simulink model "fourmasses_cvxgen"  (Simulink 7.9)
settings: Solver=ode45  StartTime=0.0  StopTime=60  RelTol=1e-3
values from neighbouring files (symbols this model uses):
  A = params.A    [cvxsolve.m]
  B = params.B    [cvxsolve.m]
  dt = 0.5    [prepFourMasses.m]    (also in prepSixMasses.m; prepSoftKS.m)
  Ed_block = Ef_block    [prepFourMasses.m]    (also in prepSixMasses.m; prepSoftKS.m)
  Ef_block = zeros(2*n,1)    [prepFourMasses.m]    (also in prepSixMasses.m; prepSoftKS.m)
  ef_block = Ef_block    [prepFourMasses.m]    (also in prepSixMasses.m; prepSoftKS.m)
  f = params.f    [cvxsolve.m]    (also in prepFourMasses.m = [0.5*ones(4,1)]; prepSixMasses.m = [.5*ones(6,1)]; prepSoftKS.m = [0.5*ones(6,1)])
  Ff = params.Ff    [cvxsolve.m]    (also in prepFourMasses.m = [[1] zeros(1,7)]; prepSixMasses.m = [[1;1] zeros(2,11)]; prepSoftKS.m = [[1;1] zeros(2,11)])
  ff = params.ff    [cvxsolve.m]    (also in prepFourMasses.m = [xmax]; prepSixMasses.m = [.3; .3]; prepSoftKS.m = [.3; .3])
  fs = params.fs    [cvxsolve.m]    (also in prepFourMasses.m = [xmax*ones(4,1) ]*100; prepSixMasses.m = [1*ones(12,1) ]*100; prepSoftKS.m = [0.3*ones(12,1) ]*100)
  Fu = params.Fu    [cvxsolve.m]    (also in prepFourMasses.m = [eye(2); -eye(2) ]; prepSixMasses.m = [eye(3); -eye(3) ]; prepSoftKS.m = [eye(3); -eye(3) ])
  Fus = [zeros(4,2)]    [prepFourMasses.m]    (also in prepSixMasses.m = [zeros(12,3)]; prepSoftKS.m = [zeros(12,3)])
  Fx = [zeros(4,8)]    [prepFourMasses.m]    (also in prepSixMasses.m = [zeros(6,12)]; prepSoftKS.m = [zeros(6,12)])
  Fxs = params.Fxs    [cvxsolve.m]    (also in prepFourMasses.m = [eye(4) zeros(4)]*100; prepSixMasses.m = [eye(6) zeros(6); prepSoftKS.m = [eye(6) zeros(6))
  m = size(B,2)    [prepFourMasses.m]    (also in prepSixMasses.m; prepSoftKS.m)
  n = size(A,1)    [prepFourMasses.m]    (also in prepSixMasses.m; prepSoftKS.m)
  Q = params.Q    [cvxsolve.m]    (also in prepFourMasses.m = eye(8); prepSixMasses.m = eye(12); prepSoftKS.m = eye(12))
  R = params.R    [cvxsolve.m]    (also in prepFourMasses.m = eye(2); prepSixMasses.m = eye(3); prepSoftKS.m = eye(3))
  T = 11    [prepFourMasses.m]    (also in prepSixMasses.m = 31; prepSoftKS.m = 10)
undefined symbols (not defined in the file or in its folder): Qf
settings Model: Creator=aeagr  LastModifiedBy=aeagr

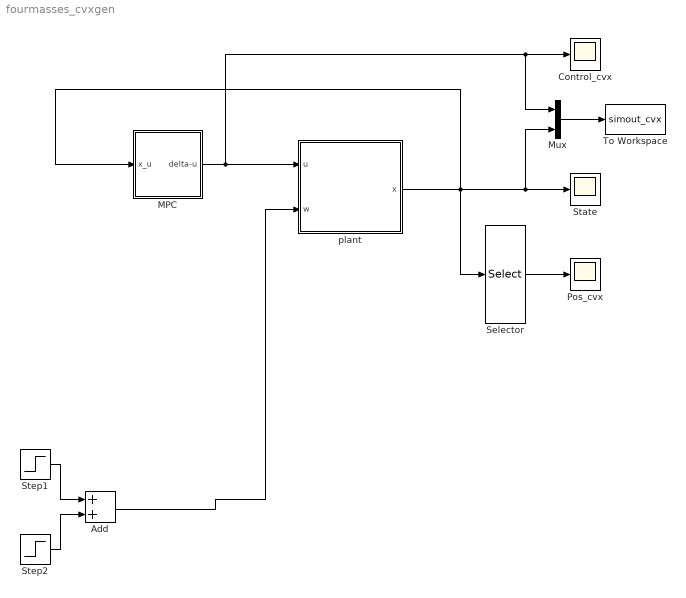
== system fourmasses_cvxgen ==
  Add : Sum
  Control_cvx : Scope
      settings: TimeRange=60  YMin=-0.5  YMax=0.45
  MPC : Subsystem  RequirementInfo={} %GIDa_b6831cb4_84cf_47ee_903b_b1a4a29acb60  TreatAsAtomicUnit=on  SystemSampleTime=dt
      settings: RTWSystemCode=Function  RTWFcnNameOpts=Use subsystem name  RTWFileNameOpts=Use subsystem name
  Mux : Mux  Inputs=2
  Pos_cvx : Scope
      settings: YMin=-0.7  YMax=0.8  SaveName=ScopeData2
  Selector : Selector  InputPortWidth=8  IndexOptions=Index vector (dialog)  Indices=[1:4]  OutputSizes=1
  State : Scope
      settings: YMin=-0.7  YMax=0.8
  Step1 : Step  Time=10  Before=zeros(4,1)  After=[0.5;0;0;0]  SampleTime=0
  Step2 : Step  Time=30  Before=zeros(4,1)  After=-[0.5;0;0;0]  SampleTime=0
  To Workspace : ToWorkspace  VariableName=simout_cvx  SampleTime=-1
  plant : Subsystem
  wires:
  MPC/1(delta-u) -> plant/1(u), Control_cvx/1, Mux/1
  plant/1(x) -> Selector/1, MPC/1(x_u), State/1, Mux/2
  Selector/1 -> Pos_cvx/1
  Add/1 -> plant/2(w)
  Step1/1 -> Add/1
  Step2/1 -> Add/2
  Mux/1 -> To Workspace/1

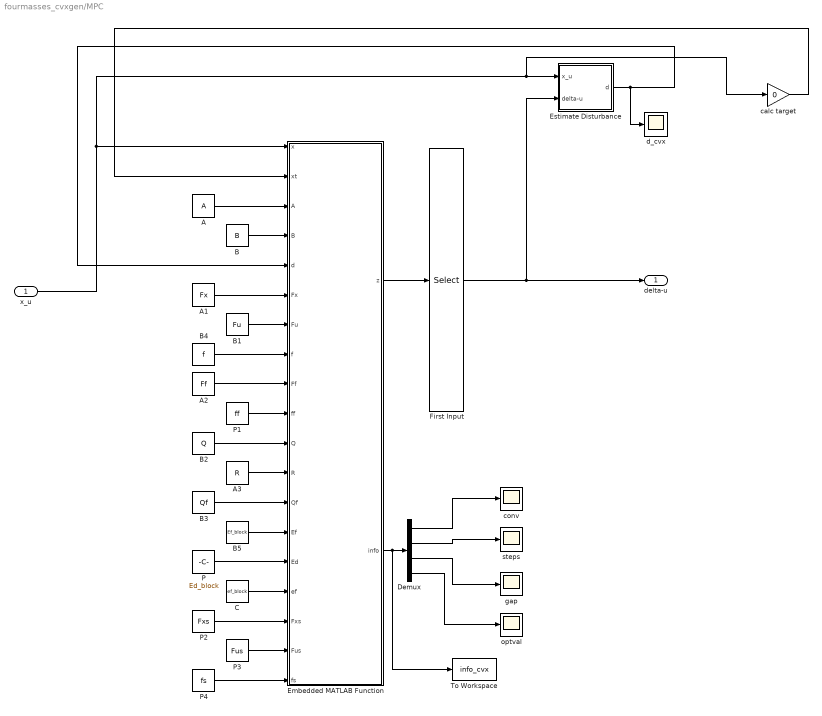
== system fourmasses_cvxgen/MPC ==
  x_u : Inport
  A : Constant  Value=A
  A1 : Constant  Value=Fx
  A2 : Constant  Value=Ff  VectorParams1D=off
  A3 : Constant  Value=R
  B : Constant  Value=B
  B1 : Constant  Value=Fu
  B2 : Constant  Value=Q
  B3 : Constant  Value=Qf
  B4 : Constant  Value=f
  B5 : Constant  Value=Ef_block
  C : Constant  Value=ef_block
  Demux : Demux
  Embedded MATLAB Function : MATLAB Function  TreatAsAtomicUnit=on
      settings: RTWFileNameOpts=Use subsystem name
  Estimate Disturbance : Subsystem
  First Input : Selector  InputPortWidth=T*(n+m)  IndexOptions=Index vector (dialog)  Indices=1:2  OutputSizes=1
  P : Constant  Value=Ed_block
  P1 : Constant  Value=ff
  P2 : Constant  Value=Fxs
  P3 : Constant  Value=Fus
  P4 : Constant  Value=fs
  To Workspace : ToWorkspace  VariableName=info_cvx  SampleTime=-1
  calc target : Gain  Gain=0
  conv : Scope
      settings: YMin=1.65436e-24  YMax=2.75e-08  SaveName=ScopeData3
  d_cvx : Scope
      settings: YMin=-0.00025  YMax=0.002  SaveName=ScopeData6
  gap : Scope
      settings: YMin=1.65436e-24  YMax=2.75e-08  SaveName=ScopeData5
  optval : Scope
      settings: YMin=1.65436e-24  YMax=2.75e-08  SaveName=ScopeData9
  steps : Scope
      settings: YMin=1.65436e-24  YMax=2.75e-08  SaveName=ScopeData4
  delta-u : Outport
  wires:
  First Input/1 -> delta-u/1, Estimate Disturbance/2(delta-u)
  Embedded MATLAB Function/1(z) -> First Input/1
  x_u/1 -> Embedded MATLAB Function/1(x), Estimate Disturbance/1(x_u), calc target/1
  B/1 -> Embedded MATLAB Function/4(B)
  A/1 -> Embedded MATLAB Function/3(A)
  B3/1 -> Embedded MATLAB Function/13(Qf)
  A3/1 -> Embedded MATLAB Function/12(R)
  B2/1 -> Embedded MATLAB Function/11(Q)
  A2/1 -> Embedded MATLAB Function/9(Ff)
  B1/1 -> Embedded MATLAB Function/7(Fu)
  A1/1 -> Embedded MATLAB Function/6(Fx)
  B4/1 -> Embedded MATLAB Function/8(f)
  P1/1 -> Embedded MATLAB Function/10(ff)
  Estimate Disturbance/1(d) -> d_cvx/1, Embedded MATLAB Function/5(d)
  calc target/1 -> Embedded MATLAB Function/2(xt)
  B5/1 -> Embedded MATLAB Function/14(Ef)
  P2/1 -> Embedded MATLAB Function/17(Fxs)
  P3/1 -> Embedded MATLAB Function/18(Fus)
  P/1 -> Embedded MATLAB Function/15(Ed)
  C/1 -> Embedded MATLAB Function/16(ef)
  P4/1 -> Embedded MATLAB Function/19(fs)
  Embedded MATLAB Function/2(info) -> Demux/1, To Workspace/1
  Demux/1 -> conv/1
  Demux/2 -> steps/1
  Demux/3 -> gap/1
  Demux/4 -> optval/1

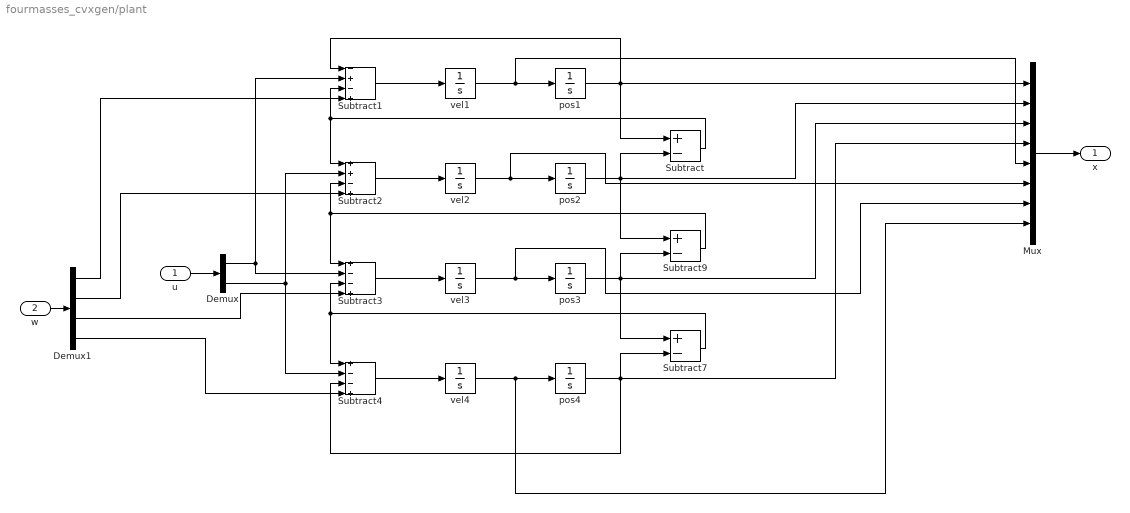
== system fourmasses_cvxgen/plant ==
  u : Inport
  w : Inport  Port=2
  Demux : Demux  Outputs=2
  Demux1 : Demux
  Mux : Mux  Inputs=8
  Subtract : Sum  Inputs=+-
  Subtract1 : Sum  Inputs=-+-+
  Subtract2 : Sum  Inputs=++-+
  Subtract3 : Sum  Inputs=+--+
  Subtract4 : Sum  Inputs=+--+
  Subtract7 : Sum  Inputs=+-
  Subtract9 : Sum  Inputs=+-
  pos{1..4} (4 alike) : Integrator
  vel{1..4} (4 alike) : Integrator
  x : Outport
  wires:
  vel1/1 -> pos1/1, Mux/5
  vel2/1 -> pos2/1, Mux/6
  vel3/1 -> pos3/1, Mux/7
  vel4/1 -> pos4/1, Mux/8
  pos1/1 -> Subtract/1, Subtract1/1, Mux/1
  pos2/1 -> Subtract/2, Subtract9/1, Mux/2
  pos3/1 -> Subtract7/1, Subtract9/2, Mux/3
  pos4/1 -> Subtract7/2, Mux/4, Subtract4/3
  Subtract/1 -> Subtract2/1, Subtract1/3
  Subtract9/1 -> Subtract3/1, Subtract2/3
  Subtract7/1 -> Subtract4/1, Subtract3/3
  Subtract4/1 -> vel4/1
  Subtract3/1 -> vel3/1
  Subtract2/1 -> vel2/1
  Subtract1/1 -> vel1/1
  Demux/1 -> Subtract1/2, Subtract3/2
  u/1 -> Demux/1
  Mux/1 -> x/1
  Demux1/3 -> Subtract3/4
  Demux1/4 -> Subtract4/4
  w/1 -> Demux1/1
  Demux1/1 -> Subtract1/4
  Demux1/2 -> Subtract2/4
  Demux/2 -> Subtract2/2, Subtract4/2

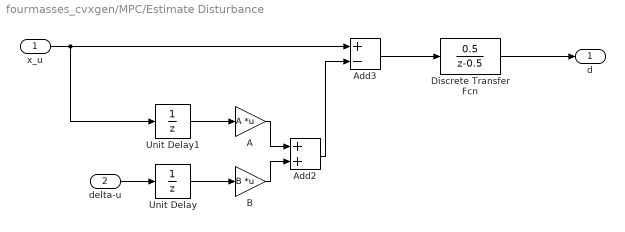
== system fourmasses_cvxgen/MPC/Estimate Disturbance ==
  x_u : Inport
  delta-u : Inport  Port=2
  A : Gain  Gain=A  Multiplication=Matrix(K*u)
  Add2 : Sum
  Add3 : Sum  Inputs=+-
  B : Gain  Gain=B  Multiplication=Matrix(K*u)
  Discrete Transfer Fcn : DiscreteTransferFcn  Numerator=[0.5]  Denominator=[1 -0.5]
  Unit Delay : UnitDelay  SampleTime=-1
  Unit Delay1 : UnitDelay  SampleTime=-1
  d : Outport
  wires:
  Unit Delay1/1 -> A/1
  Unit Delay/1 -> B/1
  A/1 -> Add2/1
  B/1 -> Add2/2
  Add2/1 -> Add3/2
  x_u/1 -> Unit Delay1/1, Add3/1
  delta-u/1 -> Unit Delay/1
  Add3/1 -> Discrete Transfer Fcn/1
  Discrete Transfer Fcn/1 -> d/1

== matlab function MPC/Embedded MATLAB Function ==
  data: x input double; xt input double; z output double; A input double; B input double; d input double; Fx input double; Fu input double; f input double; Ff input double; ff input double; Q input double; R input double; Qf input double; Ef input double; Ed input double; ef input double; Fxs input double; Fus input double; info output double; fs input double
function [z,info] = mpcsolve_simk(x,xt,A,B,d,Fx,Fu,f,Ff,ff,Q,R,Qf,Ef,Ed,ef,Fxs,Fus,fs)
%notcodegen
coder.extrinsic('cvxgenSolve')

z = zeros(210,1);
info = zeros(4,1);

% just call to the Matlab version
[z,info] = cvxgenSolve(x,xt,Q,R,Qf,A,B,d,Fx,Fu,f,Fxs,Fus,fs,Ef,Ed,ef,Ff,ff);
